simulink model "fxpdemo_filters"  (Simulink 5.0)
settings: Solver=FixedStepDiscrete  SolverMode=SingleTasking  StartTime=0.0  StopTime=1  FixedStep=0.005  RelTol=1e-3  AbsTol=1e-6
InitFcn:
  | ;
StartFcn:
  | ;
StopFcn:
  | ;
undefined symbols (not defined in the file or in its folder): NumBits1, NumBits2, Slope1, Slope2
libraries: fixpt_lib_4 x9, fixpt_lib_3p1 x1
PreSaveFcn:
  | ;
CloseFcn:
  | ;
settings Model: CovMetricSettings=d  MinMaxOverflowLogging=MinMaxAndOverflow  Creator=andyb  LastModifiedBy=andyb  ExtModeTrigMode=oneshot  ExtModeArmWhenConnect=off  ExtModeAutoUpdateStatusClock=off  LimitDataPoints=off  IntegerOverflowMsg=none  ParameterDowncastMsg=warning  ParameterOverflowMsg=warning  ParameterPrecisionLossMsg=none  RTWInlineParameters=on  RTWOptions="-aEnforceIntegerDowncast=1 -aExtMode=0 -aExtModeTesting=0 -aFoldNonRolledExpr=1 -aForceParamTrailComments=0 -aGenerateComments=0 -aGenerateReport=1 -aIgnoreCustomStorageClasses=1 -aIncDataTypeInIds=0 -aIncHierarchyInIds=0 -aInlineInvariantSignals=1 -aInlinedPrmAccess=\"Literals\" -aLocalBlockOutputs=1 -aLogVarNameModifier=\"rt_\" -aMaxRTWIdLen=31 -aPrefixModelToSubsysFcnNames=1 -aRTWVerbose=1 -aRollThreshold=5 -aShowEliminatedStatements=0"

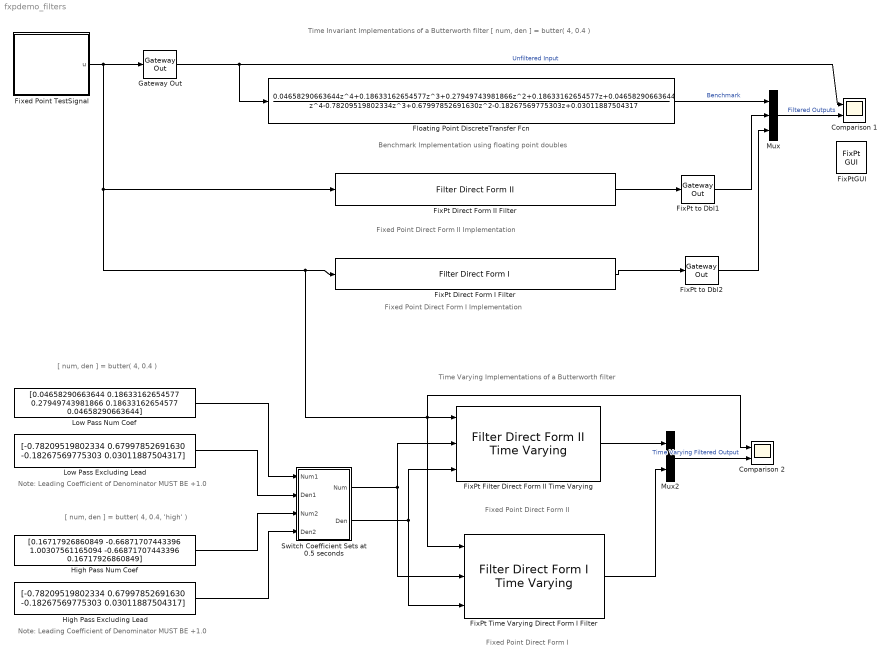
== system fxpdemo_filters ==
  note: Time Invariant
      | Implementations of a Butterworth filter
      | [ num, den ] = butter( 4, 0.4 )
  note: Benchmark Implementation using floating point doubles
  note: Note: Leading Coefficient of Denominator MUST BE +1.0
  note: Fixed Point Direct Form II
  note: Fixed Point Direct Form I Implementation
  note: Time Varying
      | Implementations of a Butterworth filter
  note: [ num, den ] = butter( 4, 0.4 )
  note: [ num, den ] = butter( 4, 0.4, 'high' )
  note: Fixed Point Direct Form I
  note: Fixed Point Direct Form II Implementation
  note: Note: Leading Coefficient of Denominator MUST BE +1.0
  Comparison 1 : Scope  NumInputPorts=2
      settings: TickLabels=on  TimeRange=1  YMin=-1~-0.8  YMax=1~0.6
  Comparison 2 : Scope  NumInputPorts=2
      settings: TickLabels=on  TimeRange=1  YMin=-1~-0.8  YMax=1~0.6  SaveName=ScopeData2
  FixPt Direct Form I Filter : fixpt_lib_4/Filters/Filter Direct Form I  NumCoefVec="[0.04658290663644  0.18633162654577 0.27949743981866  0.18633162654577 0.04658290663644]"  DenCoefVec=[-0.78209519802334 0.67997852691630 -0.18267569775303 0.03011887504317]  ICPrevOutput=0.0  ICPrevInput=0.0  DoSatur=off
  FixPt Direct Form II Filter : fixpt_lib_4/Filters/Filter Direct Form II  NumCoefVec="[0.04658290663644  0.18633162654577 0.27949743981866  0.18633162654577 0.04658290663644]"  DenCoefVec=[-0.78209519802334 0.67997852691630 -0.18267569775303 0.03011887504317]  vinit=0.0  DoSatur=off
  FixPt Filter Direct Form II Time Varying : fixpt_lib_4/Filters/Filter Direct Form II Time Varying  vinit=0.0  DoSatur=off
  FixPt Time Varying Direct Form I Filter : fixpt_lib_4/Filters/Filter Direct Form I Time Varying  ICPrevOutput=0.0  ICPrevInput=0.0  DoSatur=off
  FixPt to Dbl1 : fixpt_lib_4/Data Type/Gateway Out  OutRealWorld=Real World Value  OutBuiltInType=double  DoSatur=off
  FixPt to Dbl2 : fixpt_lib_4/Data Type/Gateway Out  OutRealWorld=Real World Value  OutBuiltInType=double  DoSatur=off
  FixPtGUI : fixpt_lib_3p1/FixPt GUI
  Fixed Point TestSignal : Subsystem
      mask Display: fprintf('Sine Waves\n0.5 @ 2Hz\nplus\n0.5 @ 80Hz')
  Floating Point DiscreteTransfer Fcn : DiscreteTransferFcn  Numerator="[0.04658290663644  0.18633162654577 0.27949743981866  0.18633162654577 0.04658290663644]"  Denominator=[1.00000000000000 -0.78209519802334 0.67997852691630 -0.18267569775303 0.03011887504317]  SampleTime=-1
  Gateway Out : fixpt_lib_4/Data Type/Gateway Out  OutRealWorld=Real World Value  OutBuiltInType=double  DoSatur=off
  High Pass Excluding Lead : Constant  Value="[-0.78209519802334   0.67997852691630  -0.18267569775303 0.03011887504317]"  ShowAdditionalParam=on  OutDataTypeMode=Specify via dialog  ConRadixGroup=Best Precision: Vector-wise  OutScaling=2^-15
  High Pass Num Coef : Constant  Value="[0.16717926860849  -0.66871707443396   1.00307561165094  -0.66871707443396 0.16717926860849]"  ShowAdditionalParam=on  OutDataTypeMode=Specify via dialog  ConRadixGroup=Best Precision: Vector-wise  OutScaling=2^-14
  Low Pass Excluding Lead : Constant  Value=[-0.78209519802334 0.67997852691630 -0.18267569775303 0.03011887504317]  ShowAdditionalParam=on  OutDataTypeMode=Specify via dialog  ConRadixGroup=Best Precision: Vector-wise  OutScaling=2^-15
  Low Pass Num Coef : Constant  Value="[0.04658290663644 0.18633162654577 0.27949743981866  0.18633162654577 0.04658290663644]"  ShowAdditionalParam=on  OutDataTypeMode=Specify via dialog  ConRadixGroup=Best Precision: Vector-wise  OutScaling=2^-16
  Mux : Mux  Inputs=3
  Mux2 : Mux  Inputs=2
  Switch Coefficient Sets at 0.5 seconds : Subsystem
  wires:
  Fixed Point TestSignal/1(u) -> Gateway Out/1, Comparison 2/1, FixPt Filter Direct Form II Time Varying/1, FixPt Time Varying Direct Form I Filter/1, FixPt Direct Form I Filter/1, FixPt Direct Form II Filter/1
  Mux/1 -> Comparison 1/2  "Filtered Outputs"
  Floating Point DiscreteTransfer Fcn/1 -> Mux/1  "Benchmark"
  Gateway Out/1 -> Floating Point DiscreteTransfer Fcn/1, Comparison 1/1  "Unfiltered Input"
  FixPt Filter Direct Form II Time Varying/1 -> Mux2/1
  Mux2/1 -> Comparison 2/2  "Time Varying Filtered Output"
  FixPt Time Varying Direct Form I Filter/1 -> Mux2/2
  Low Pass Num Coef/1 -> Switch Coefficient Sets at 0.5 seconds/1(Num1)
  Low Pass Excluding Lead/1 -> Switch Coefficient Sets at 0.5 seconds/2(Den1)
  High Pass Num Coef/1 -> Switch Coefficient Sets at 0.5 seconds/3(Num2)
  High Pass Excluding Lead/1 -> Switch Coefficient Sets at 0.5 seconds/4(Den2)
  Switch Coefficient Sets at 0.5 seconds/1(Num) -> FixPt Filter Direct Form II Time Varying/2, FixPt Time Varying Direct Form I Filter/2
  Switch Coefficient Sets at 0.5 seconds/2(Den) -> FixPt Filter Direct Form II Time Varying/3, FixPt Time Varying Direct Form I Filter/3
  FixPt Direct Form II Filter/1 -> FixPt to Dbl1/1
  FixPt Direct Form I Filter/1 -> FixPt to Dbl2/1
  FixPt to Dbl1/1 -> Mux/2
  FixPt to Dbl2/1 -> Mux/3

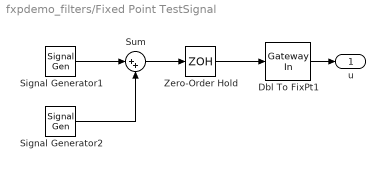
== system fxpdemo_filters/Fixed Point TestSignal ==
  Dbl To FixPt1 : fixpt_lib_4/Data Type/Gateway In  InRealWorld=Real World Value  OutputDataTypeScalingMode=Specify via dialog  OutDataType=sfix(16)  OutScaling=2^(-15)  DoSatur=on
      settings: LockScale=on
  Signal Generator1 : SignalGenerator  Amplitude=0.5  Frequency=2
  Signal Generator2 : SignalGenerator  Amplitude=0.5  Frequency=80
  Sum : Sum  Inputs=|++  SaturateOnIntegerOverflow=on  InputSameDT=on
  Zero-Order Hold : ZeroOrderHold  SampleTime=0.005
  u : Outport
  wires:
  Zero-Order Hold/1 -> Dbl To FixPt1/1
  Sum/1 -> Zero-Order Hold/1
  Signal Generator1/1 -> Sum/1
  Signal Generator2/1 -> Sum/2
  Dbl To FixPt1/1 -> u/1

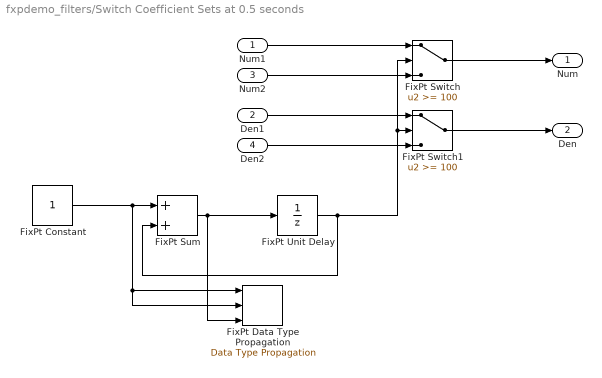
== system fxpdemo_filters/Switch Coefficient Sets at 0.5 seconds ==
  Num1 : Inport
  Den1 : Inport  Port=2
  Num2 : Inport  Port=3
  Den2 : Inport  Port=4
  FixPt Constant : Constant  ShowAdditionalParam=on  OutDataTypeMode=Specify via dialog  OutDataType=ufix(16)
  FixPt Data Type Propagation : fixpt_lib_4/Data Type/Data Type Propagation  PropDataType=sfix(16)  IfRefDouble=double  IfRefSingle=single  IsSigned=IsSigned1 or IsSigned2  NumBitsBase=max([NumBits1 NumBits2])  NumBitsMult=1  NumBitsAdd=0  NumBitsAllowFinal=1:128  PropScaling=2^-10  ValuesUsedBestPrec=[5 -7]  SlopeBase=min([Slope1 Slope2])  SlopeMult=1  SlopeAdd=0  BiasBase=Bias1  BiasMult=1  BiasAdd=0
  FixPt Sum : Sum  ShowAdditionalParam=on  OutScaling=2^-10
  FixPt Switch : Switch  Threshold=100  ShowAdditionalParam=on
  FixPt Switch1 : Switch  Threshold=100  ShowAdditionalParam=on
  FixPt Unit Delay : UnitDelay  X0=0.0  SampleTime=-1
  Num : Outport
  Den : Outport  Port=2
  wires:
  FixPt Constant/1 -> FixPt Sum/1, FixPt Data Type Propagation/1, FixPt Data Type Propagation/2
  FixPt Sum/1 -> FixPt Unit Delay/1, FixPt Data Type Propagation/3
  FixPt Unit Delay/1 -> FixPt Sum/2, FixPt Switch/2, FixPt Switch1/2
  Num1/1 -> FixPt Switch/1
  FixPt Switch/1 -> Num/1
  Num2/1 -> FixPt Switch/3
  Den1/1 -> FixPt Switch1/1
  FixPt Switch1/1 -> Den/1
  Den2/1 -> FixPt Switch1/3
